simulink model "Lab1"  (R2023b)
settings: Solver=VariableStepAuto  StartTime=0.0  StopTime=inf  RelTol=1e-3
undefined symbols (not defined in the file): designMultirateFIR, Fs, ip, usb
libraries: plutoradiolib x1, dspsnks4 x1, dspsigops x1, dspfdesign x1, dspmlti4 x1
settings Model: Creator=shreejiths  LastModifiedBy=LEE
settings DebuggingCC: UnconnectedInputMsg=warning  UnconnectedOutputMsg=warning  UnconnectedLineMsg=warning
settings ModelReferenceCC: EnableRefExpFcnMdlSchedulingChecks=on
settings RTWCC: DLArmComputeVersion=19.05

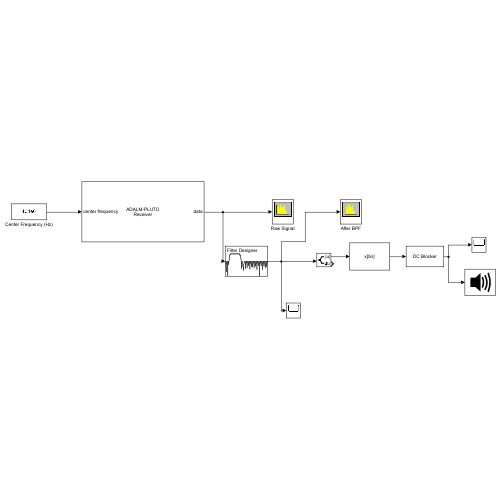
[thumbnail: Simulink's stored preview of the top-level diagram]
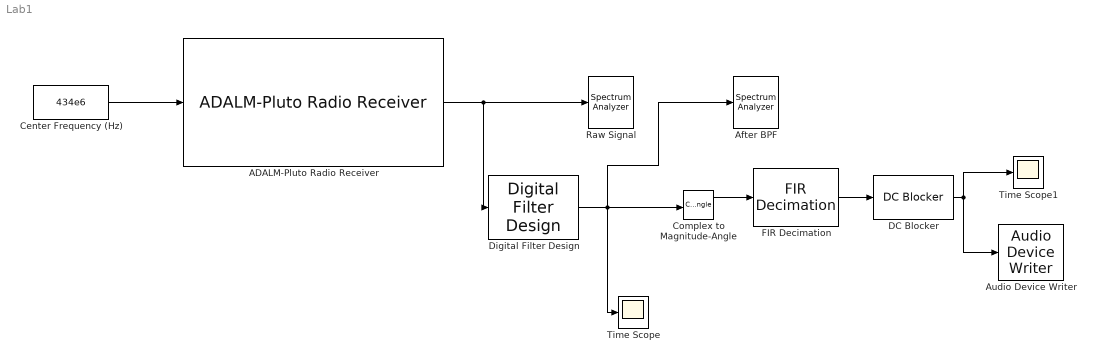
== system Lab1 ==
  ADALM-Pluto Radio Receiver : plutoradiolib/ADALM-Pluto Radio Receiver  RadioID=usb:0  uri=ip:10.0.0.200  CenterFrequencySource=Input Port  CenterFrequency=2.4e9  GainSource=AGC Slow Attack  GainSourceBlock=Dialog  Gain=40  ChannelMapping=1  BasebandSampleRate=2.4e5  OutputDataType=single  SamplesPerFrame=3660  OverflowOutputPort=off  EnableBurstMode=off  NumFramesInBurst=1  ShowAdvancedProperties=off  UseCustomFilter=off  filtPathRates=[737280000 11520000 3840000 1920000 960000 240000]  filtCoefficients=[-192 82 85 -215 228 -102 -110 290 -318 145 160 -426 471 -215 -238 633 -697 318 349 -923 1009 -457 -498 1309 -1423 640 693 -1812 1959 -876 -945 2458 -2647 1180 1268 -3290 3534 -1572 -1688 4375 -4698 2091 2247 -5836 6284 -2807 -3031 7918 -8588 3870 4225 -11182 12324 -5662 -6330 17255 -19735 9507 11312 -33568 43355 -25227 -42139 305542 305542 -42139 -25227 43355 -33568 11312 9507 -19735 17255 -6330 -5662 12324 -11182 4225 3870 -8588 7918 -3031 -2807 6284 -5836 2247 2091 -4698 4375 -1688 -1572 3534 -3290 1268 1180 -2647 2458 -945 -876 1959 -1812 693 640 -1423 1309 -498 -457 1009 -923 349 318 -697 633 -238 -215 471 -426 160 145 -318 290 -110 -102 228 -215 85 82 -192]  filtCoefficientSize=128  filtDecimInterpFactor=4  filtGain=-12  filtRFBandwidth=18000000  filterConfigStruct=struct()  EnableQuadratureCorrection=on  EnableRFDCCorrection=on  EnableBasebandDCCorrection=on  FrequencyCorrection=0  OverrideSampleTime=off  SampleTime=0.02  DataTimeout=Inf  ENSMPinControlMode=None  BISTLoopbackMode=Disabled  BISTToneInject=Disabled  BISTSignalGen=PRBS  BISTToneFreq=Fs/32  BISTToneLevel=0
  After BPF : SpectrumAnalyzer  WindowPosition=[1.000000,41.000000,1728.000000,1089.000000,]  ScopeFrameLocation=window  SampleRate=4000000  AxesScaling=Manual  Span=6000000  StartFrequency=-2000000  StopFrequency=2000000  FrequencyResolutionMethod=Number of frequency bands  AveragingMethod=Exponential  YLimits=[-175.89512889,-49.01606597]  ColorLimits=[-1.4480614138038987448,14.840270108115898751]  AxesLayout=Horizontal  ExpandToolstrip=on  DefaultConfigurationName=spbscopes.SpectrumAnalyzerBlockCfg  IsFrequencyInputMode=0  FrequencyVectorPort=0  FrequencyVectorFromPort=0  FrequencyInputRBWPort=0  FrequencyInputRBWFromPort=0
  Audio Device Writer : dspsnks4/Audio Device Writer  Driver=DirectSound  Device=扬声器 (Realtek(R) Audio)  InheritSampleRate=on  SampleRate=44100  BitDepth=16-bit integer  BufferSize=4096  NumBuffers=10  DefaultOutputChannelMapping=on  OutputChannelMapping=1:2  OutputNumUnderrunSamples=off  DriverIdx=1  DeviceWarnFlag=''
  Center Frequency (Hz) : Constant  Value=434e6  VectorParams1D=off
  Complex to Magnitude-Angle : ComplexToMagnitudeAngle
  DC Blocker : dspsigops/DC Blocker  Algorithm=IIR  NormalizedBandwidth=0.001  Length=8  Order=6  SimulateUsing=Code generation
      settings: LibrarySourceBlock=commfilt2/DC Blocker
  Digital Filter Design : dspfdesign/Digital Filter Design  mwdsp_browser_bugfix_var=off
  FIR Decimation : dspmlti4/FIR Decimation  FilterSource=Auto  h=designMultirateFIR(1,2)  D=5  filtStruct=Direct form  FilterObject=FDECIM  InputProcessing=Columns as channels (frame based)  framing=Enforce single-rate processing  AllowArbitraryInputLength=off  inputOffset=0  outputBufInitCond=0  roundingMode=Floor  overflowMode=off  firstCoeffDataTypeStr=Inherit: Same word length as input  firstCoeffMin=[]  firstCoeffMax=[]  firstCoeffLastDataTypeStr=Inherit: Same word length as input  outputDataTypeStr=Inherit: Same as accumulator  outputMin=[]  outputMax=[]  outputLastDataTypeStr=Inherit: Same as accumulator
  Raw Signal : SpectrumAnalyzer  WindowPosition=[1.000000,-45.000000,1728.000000,1089.000000,]  ScopeFrameLocation=window  SampleRate=4000000  AxesScaling=Manual  Span=6000000  StartFrequency=-2000000  StopFrequency=2000000  FrequencyResolutionMethod=Number of frequency bands  AveragingMethod=Exponential  YLimits=[-85.48264357,-41.97045773]  ColorLimits=[-1.4480614138038987448,14.840270108115898751]  AxesLayout=Horizontal  DefaultConfigurationName=spbscopes.SpectrumAnalyzerBlockCfg  IsFrequencyInputMode=0  FrequencyVectorPort=0  FrequencyVectorFromPort=0  FrequencyInputRBWPort=0  FrequencyInputRBWFromPort=0
  Time Scope : Scope
  Time Scope1 : Scope
  wires:
  Center Frequency (Hz)/1 -> ADALM-Pluto Radio Receiver/1
  ADALM-Pluto Radio Receiver/1 -> Digital Filter Design/1, Raw Signal/1
  Digital Filter Design/1 -> Time Scope/1, Complex to Magnitude-Angle/1, After BPF/1
  Complex to Magnitude-Angle/1 -> FIR Decimation/1
  FIR Decimation/1 -> DC Blocker/1
  DC Blocker/1 -> Audio Device Writer/1, Time Scope1/1
